simulink library "AP_Lib_rev"  (R2013a)
settings: Solver=ode45  StartTime=0.0  StopTime=10.0  RelTol=1e-3
undefined symbols (not defined in the file): intLim
settings Model: Creator=bpotter  LastModifiedBy=bpotter

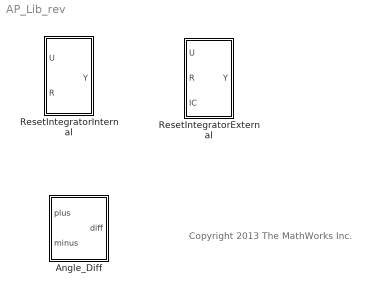
== system AP_Lib_rev ==
  note: Copyright 2013 The MathWorks Inc.
  Angle_Diff : Subsystem
      settings: AttributesFormatString=-180 deg to +180 deg range
  ResetIntegratorExternal : Subsystem  mask(SLCI_Level_Reset_Integrator){K=1.0, Ts=1/40, UL=intLim}
      mask prompts: K "Gain value:"; Ts "Sample time (-1 for inherited):"; UL "Symmetrical saturation limit:"
      mask help: Level reset integrator using Forward Euler method. This masked subsystem implements the functional behavior of Simulink's Descrete-Time Integrator block using Simulink Code Inspector supported blocks.
      settings: AttributesFormatString=K = %<K>\n-%<UL> to %<UL>
      mask Display: fprintf('K Ts\n____\nz-1')
  ResetIntegratorInternal : Subsystem  RequirementInfo={} %GIDa_205543a7_57f5_4e95_8a94_c6cb06cf5949  mask(SLCI_Level_Reset_Integrator){K=1.0, Ts=1/40, IC=0, UL=intLim}
      mask prompts: K "Gain value:"; Ts "Sample time (-1 for inherited):"; IC "Initial condition:"; UL "Symmetric saturation limit:"
      mask help: Level reset integrator using Forward Euler method. This masked subsystem implements the functional behavior of Simulink's Descrete-Time Integrator block using Simulink Code Inspector supported blocks.
      settings: AttributesFormatString="K =  %<K>\\n-%<UL> to %<UL>\\nIC = %<IC>"
      mask Display: fprintf('K Ts\n____\nz-1')

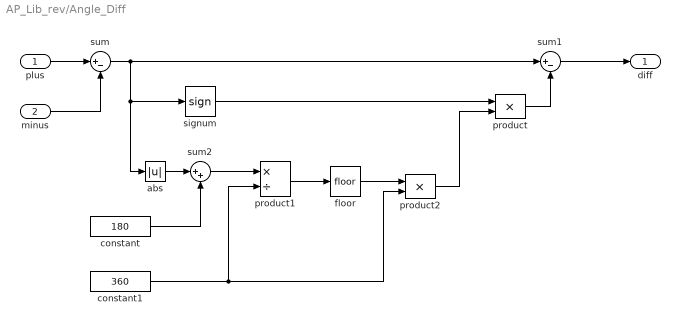
== system AP_Lib_rev/Angle_Diff ==
  plus : Inport  OutDataTypeStr=double
  minus : Inport  Port=2  OutDataTypeStr=double
  abs : Abs  ZeroCross=off
  constant : Constant  Value=180
  constant1 : Constant  Value=360
  floor : Rounding
  product : Product  RndMeth=Zero  InputSameDT=on  OutDataTypeStr=Inherit: Same as first input
  product1 : Product  Inputs=*/  RndMeth=Zero  InputSameDT=on  OutDataTypeStr=Inherit: Same as first input
  product2 : Product  RndMeth=Zero  InputSameDT=on  OutDataTypeStr=Inherit: Same as first input
  signum : Signum  ZeroCross=off
  sum : Sum  Inputs=|+-  RndMeth=Zero  InputSameDT=on  OutDataTypeStr=Inherit: Same as first input
  sum1 : Sum  Inputs=|+-  RndMeth=Zero  InputSameDT=on  OutDataTypeStr=Inherit: Same as first input
  sum2 : Sum  Inputs=|++  RndMeth=Zero  InputSameDT=on  OutDataTypeStr=Inherit: Same as first input
  diff : Outport
  wires:
  sum2/1 -> product1/1
  product/1 -> sum1/2
  product2/1 -> product/2
  signum/1 -> product/1
  sum1/1 -> diff/1
  constant/1 -> sum2/2
  floor/1 -> product2/1
  minus/1 -> sum/2
  plus/1 -> sum/1
  sum/1 -> signum/1, abs/1, sum1/1
  abs/1 -> sum2/1
  constant1/1 -> product1/2, product2/2
  product1/1 -> floor/1

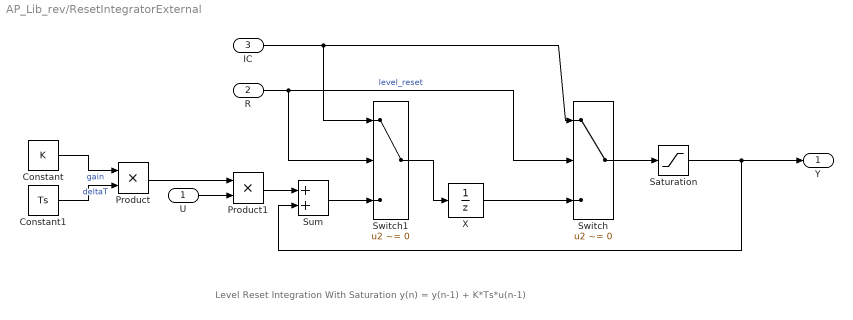
== system AP_Lib_rev/ResetIntegratorExternal ==
  note: Level Reset Integration With Saturation
      | y(n) = y(n-1) + K*Ts*u(n-1)
  U : Inport
  R : Inport  Port=2
  IC : Inport  Port=3
  Constant : Constant  Value=K
  Constant1 : Constant  Value=Ts
  Product : Product  RndMeth=Zero
  Product1 : Product  RndMeth=Zero
  Saturation : Saturate  UpperLimit=UL  LowerLimit=-UL
  Sum : Sum
  Switch : Switch  Criteria=u2 ~= 0
  Switch1 : Switch  Criteria=u2 ~= 0
  X : UnitDelay  SampleTime=Ts
  Y : Outport
  wires:
  R/1 -> Switch1/2, Switch/2  "level_reset"
  Sum/1 -> Switch1/3
  Switch1/1 -> X/1
  Constant/1 -> Product/1  "gain"
  Constant1/1 -> Product/2  "deltaT"
  Product/1 -> Product1/1
  U/1 -> Product1/2
  Product1/1 -> Sum/1
  IC/1 -> Switch1/1, Switch/1
  Switch/1 -> Saturation/1
  Saturation/1 -> Y/1, Sum/2
  X/1 -> Switch/3

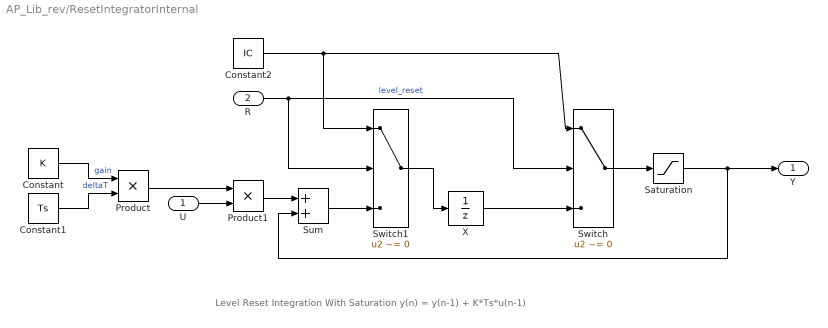
== system AP_Lib_rev/ResetIntegratorInternal ==
  note: Level Reset Integration With Saturation
      | y(n) = y(n-1) + K*Ts*u(n-1)
  U : Inport
  R : Inport  Port=2
  Constant : Constant  Value=K
  Constant1 : Constant  Value=Ts
  Constant2 : Constant  Value=IC
  Product : Product  RndMeth=Zero
  Product1 : Product  RndMeth=Zero
  Saturation : Saturate  UpperLimit=UL  LowerLimit=-UL
  Sum : Sum
  Switch : Switch  Criteria=u2 ~= 0
  Switch1 : Switch  Criteria=u2 ~= 0
  X : UnitDelay  InitialCondition=IC  SampleTime=Ts
  Y : Outport
  wires:
  Switch/1 -> Saturation/1
  Constant2/1 -> Switch/1, Switch1/1
  Product1/1 -> Sum/1
  U/1 -> Product1/2
  Product/1 -> Product1/1
  Constant1/1 -> Product/2  "deltaT"
  Constant/1 -> Product/1  "gain"
  Switch1/1 -> X/1
  Sum/1 -> Switch1/3
  R/1 -> Switch/2, Switch1/2  "level_reset"
  Saturation/1 -> Sum/2, Y/1
  X/1 -> Switch/3
